simulink library "lib_transmission2"  (Simulink 10.1)
settings: Solver=VariableStepAuto  StartTime=0.0  StopTime=10.0  RelTol=1e-3
undefined symbols (not defined in the file or in its folder): cyc_mph, fc_map_spd, fc_max_trq, fc_spd_scale, fc_trq_scale, fd_inertia, fd_loss, fd_ratio, gb_gear_number_lookup, gb_gears_num, gb_inertia, gb_loss_const, gb_loss_input_spd_coeff, gb_loss_input_trq_coeff, gb_loss_output_spd_coeff, gb_loss_output_trq_coeff, gb_num_init, gb_ratio, gb_shift_delay, gb_spd_scale, gb_trq_scale, htc_inertia, htc_k_adv, htc_k_adv_coast, htc_lockup, htc_lockup_load, htc_lockup_spd, htc_lu_gear_range, htc_max_coast_tr, htc_min_coast_tr, htc_pump_loss_spd, htc_pump_loss_trq_lockup, htc_pump_loss_trq_unlock, htc_sr, htc_sr_coast, htc_tr, htc_tr_coast, htc_unlock_spd, mc_map_spd, mc_max_trq, mc_overtrq_factor, mc_spd_scale, mc_trq_scale, tc_loss, tc_mc_to_fc_ratio, tx_eff_map, tx_map_spd, tx_map_trq, tx_pg_r, tx_pg_s, tx_speed_dep, vc_clutch_bool, vc_idle_spd, vc_launch_spd, wh_radius
undefined symbols (not defined in the file): gb_dnshift_load, gb_dnshift_spd, gb_map_spd_out, gb_map_trq_in, gb_map_trq_out, gb_upshift_load, gb_upshift_spd, logFlag
libraries: lib_controls x1, lib_etc x1, lib_controls2 x1, lib_transmission x1
(part 11 of 17)

== system lib_transmission2/torque coupler <tc>/tc model & interface/tc model ==
  "torque and speed req'd at output side of torque coupler (Nm), (rad/s)" : Inport
  "torque and speed avail. at main input (Nm), (rad/s)" : Inport  Port=2
  "torque and speed avail. at motor input to tc (Nm), (rad/s)" : Inport  Port=3
  Block NOTES : Subsystem
      mask Display: disp('Block\nNOTES')
  Demux : Demux  Outputs=2
  Demux1 : Demux  Outputs=2
  Demux2 : Demux  Outputs=2
  MinMax : MinMax  Inputs=2
  MinMax1 : MinMax  Inputs=2
  Mux : Mux  Inputs=2
  Mux1 : Mux  Inputs=2
  Mux2 : Mux  Inputs=2
  Product : Product  Inputs=1  SaturateOnIntegerOverflow=on
  Product1 : Product  Inputs=1  SaturateOnIntegerOverflow=on
  effect of motor torque at output of tc (Nm) : Gain  Gain=tc_mc_to_fc_ratio  SaturateOnIntegerOverflow=on
  enhancedToWorkspace : Subsystem  TreatAsAtomicUnit=on  mask(enhancedToWorkspace){generalName=generalName, specificName=spd_out_r, logFlag=logFlag}
      mask prompts: generalName "General Name [char-evaluated]"; specificName "Specific Name [char-literal]"; logFlag "Enable flag (1=on,0=off)"
      mask help: A wrapper for the Simulink "To Workspace" block that allows you to evaluate the name of the variable to log to workspace. This is useful to avoid the double logging errors that occur when you pull in two library models that attempt to log to the same variable.
      mask init:
      | enhancedToWsMaker
      settings: CopyFcn=breakLinkCopyFcn  ParentCloseFcn=breakLinkParCloseFcn
      mask Help:
      | <h2>Enhanced To Workspace Block</h2>
      | <h3>Parameters</h3>
      | <UL>
      | <li><b>General Name:</b> This is the more general name of the variable. Variables are saved to the workspace as <i>generalName_specificName</i>. Note that this is an evaluated variable. If you would like to type in the value directly, it must be surrounded with single quotes. Otherwise you can input the name of a variable containing a char string.</li>
      | <li><b>Specific Name:</b> This is the specific name of the variable. Note that this is input as a char literal (i.e., you don't need quotes).</li>
      | <li><b>Enable Flag:</b> This flag should have the value of 0 or 1. If 0, the variable will not be logged to the workspace. If 1, the variable will be logged. This is done so that variable logging can be turned off to improve speed.</li>
      | </ul>
      | <h3>Overview</h3>
      | <p>The enhanced to workspace block was put together to allow one to dynamically resolve variable names at run time in simulink. This is most powerful when used in conjunction with a masked subsystem to allow multiple instances of that masked subsytem to be used in the same model. The strategy is to set the generalName in the block mask which will allow the block to change the general name for all variable logging on the fly.
      | <h3>Helper Files</h3>
      | <p>Three m-files are required by the enhancedToWorkspace block. These files are located in the &lt; ADVISOR root &gt;/GUI directory :
      | <ul>
      | <li><i>enhancedToWsMaker.m</i> This file runs the mask initialization for the block</li>
      | <li><i>breakLinkCopyFcn.m</i> This file is used by the block callback when the simulink block is copied. It is necessary to break the link to the enhancedToWorkspace similar to the To Workspace block in order for it to be able to configure itself. (Try copying simulink's To Workspace block--it is impossible to make a link)</li>
      | <li><i>breakLinkParCloseFcn.m</i> This file is similar to the breakLinkCopyFcn and is used when a parent system is closed</li>
      | </ul>
      | <hr>
      | 
      | <p>Created 2003-Jan-21, Michael Patrick O'Keefe, NREL</p>
      | 
      | <!--
      | <VARDEF>
      | <H3>var_name</H3>
      | <UL>
      | <LI><B>data type</B> data type here</LI>
      | <LI><B>units</B> units here</LI>
      | <LI><B>vehicle type</B> vehicle type here</LI>
      | <LI><B>description</B> description here</LI>
      | </UL>
      | </VARDEF>
      | -->
      mask Display: disp([generalName,'_',specificName])
  enhancedToWorkspace1 : Subsystem  TreatAsAtomicUnit=on  mask(enhancedToWorkspace){generalName=generalName, specificName=trq_out_r, logFlag=logFlag}
      mask prompts: generalName "General Name [char-evaluated]"; specificName "Specific Name [char-literal]"; logFlag "Enable flag (1=on,0=off)"
      mask help: A wrapper for the Simulink "To Workspace" block that allows you to evaluate the name of the variable to log to workspace. This is useful to avoid the double logging errors that occur when you pull in two library models that attempt to log to the same variable.
      mask init:
      | enhancedToWsMaker
      settings: CopyFcn=breakLinkCopyFcn  ParentCloseFcn=breakLinkParCloseFcn
      mask Help:
      | <h2>Enhanced To Workspace Block</h2>
      | <h3>Parameters</h3>
      | <UL>
      | <li><b>General Name:</b> This is the more general name of the variable. Variables are saved to the workspace as <i>generalName_specificName</i>. Note that this is an evaluated variable. If you would like to type in the value directly, it must be surrounded with single quotes. Otherwise you can input the name of a variable containing a char string.</li>
      | <li><b>Specific Name:</b> This is the specific name of the variable. Note that this is input as a char literal (i.e., you don't need quotes).</li>
      | <li><b>Enable Flag:</b> This flag should have the value of 0 or 1. If 0, the variable will not be logged to the workspace. If 1, the variable will be logged. This is done so that variable logging can be turned off to improve speed.</li>
      | </ul>
      | <h3>Overview</h3>
      | <p>The enhanced to workspace block was put together to allow one to dynamically resolve variable names at run time in simulink. This is most powerful when used in conjunction with a masked subsystem to allow multiple instances of that masked subsytem to be used in the same model. The strategy is to set the generalName in the block mask which will allow the block to change the general name for all variable logging on the fly.
      | <h3>Helper Files</h3>
      | <p>Three m-files are required by the enhancedToWorkspace block. These files are located in the &lt; ADVISOR root &gt;/GUI directory :
      | <ul>
      | <li><i>enhancedToWsMaker.m</i> This file runs the mask initialization for the block</li>
      | <li><i>breakLinkCopyFcn.m</i> This file is used by the block callback when the simulink block is copied. It is necessary to break the link to the enhancedToWorkspace similar to the To Workspace block in order for it to be able to configure itself. (Try copying simulink's To Workspace block--it is impossible to make a link)</li>
      | <li><i>breakLinkParCloseFcn.m</i> This file is similar to the breakLinkCopyFcn and is used when a parent system is closed</li>
      | </ul>
      | <hr>
      | 
      | <p>Created 2003-Jan-21, Michael Patrick O'Keefe, NREL</p>
      | 
      | <!--
      | <VARDEF>
      | <H3>var_name</H3>
      | <UL>
      | <LI><B>data type</B> data type here</LI>
      | <LI><B>units</B> units here</LI>
      | <LI><B>vehicle type</B> vehicle type here</LI>
      | <LI><B>description</B> description here</LI>
      | </UL>
      | </VARDEF>
      | -->
      mask Display: disp([generalName,'_',specificName])
  enhancedToWorkspace2 : Subsystem  TreatAsAtomicUnit=on  mask(enhancedToWorkspace){generalName=generalName, specificName=pwr_in_a, logFlag=logFlag}
      mask prompts: generalName "General Name [char-evaluated]"; specificName "Specific Name [char-literal]"; logFlag "Enable flag (1=on,0=off)"
      mask help: A wrapper for the Simulink "To Workspace" block that allows you to evaluate the name of the variable to log to workspace. This is useful to avoid the double logging errors that occur when you pull in two library models that attempt to log to the same variable.
      mask init:
      | enhancedToWsMaker
      settings: CopyFcn=breakLinkCopyFcn  ParentCloseFcn=breakLinkParCloseFcn
      mask Help:
      | <h2>Enhanced To Workspace Block</h2>
      | <h3>Parameters</h3>
      | <UL>
      | <li><b>General Name:</b> This is the more general name of the variable. Variables are saved to the workspace as <i>generalName_specificName</i>. Note that this is an evaluated variable. If you would like to type in the value directly, it must be surrounded with single quotes. Otherwise you can input the name of a variable containing a char string.</li>
      | <li><b>Specific Name:</b> This is the specific name of the variable. Note that this is input as a char literal (i.e., you don't need quotes).</li>
      | <li><b>Enable Flag:</b> This flag should have the value of 0 or 1. If 0, the variable will not be logged to the workspace. If 1, the variable will be logged. This is done so that variable logging can be turned off to improve speed.</li>
      | </ul>
      | <h3>Overview</h3>
      | <p>The enhanced to workspace block was put together to allow one to dynamically resolve variable names at run time in simulink. This is most powerful when used in conjunction with a masked subsystem to allow multiple instances of that masked subsytem to be used in the same model. The strategy is to set the generalName in the block mask which will allow the block to change the general name for all variable logging on the fly.
      | <h3>Helper Files</h3>
      | <p>Three m-files are required by the enhancedToWorkspace block. These files are located in the &lt; ADVISOR root &gt;/GUI directory :
      | <ul>
      | <li><i>enhancedToWsMaker.m</i> This file runs the mask initialization for the block</li>
      | <li><i>breakLinkCopyFcn.m</i> This file is used by the block callback when the simulink block is copied. It is necessary to break the link to the enhancedToWorkspace similar to the To Workspace block in order for it to be able to configure itself. (Try copying simulink's To Workspace block--it is impossible to make a link)</li>
      | <li><i>breakLinkParCloseFcn.m</i> This file is similar to the breakLinkCopyFcn and is used when a parent system is closed</li>
      | </ul>
      | <hr>
      | 
      | <p>Created 2003-Jan-21, Michael Patrick O'Keefe, NREL</p>
      | 
      | <!--
      | <VARDEF>
      | <H3>var_name</H3>
      | <UL>
      | <LI><B>data type</B> data type here</LI>
      | <LI><B>units</B> units here</LI>
      | <LI><B>vehicle type</B> vehicle type here</LI>
      | <LI><B>description</B> description here</LI>
      | </UL>
      | </VARDEF>
      | -->
      mask Display: disp([generalName,'_',specificName])
  enhancedToWorkspace3 : Subsystem  TreatAsAtomicUnit=on  mask(enhancedToWorkspace){generalName=generalName, specificName=trq_out_a, logFlag=logFlag}
      mask prompts: generalName "General Name [char-evaluated]"; specificName "Specific Name [char-literal]"; logFlag "Enable flag (1=on,0=off)"
      mask help: A wrapper for the Simulink "To Workspace" block that allows you to evaluate the name of the variable to log to workspace. This is useful to avoid the double logging errors that occur when you pull in two library models that attempt to log to the same variable.
      mask init:
      | enhancedToWsMaker
      settings: CopyFcn=breakLinkCopyFcn  ParentCloseFcn=breakLinkParCloseFcn
      mask Help:
      | <h2>Enhanced To Workspace Block</h2>
      | <h3>Parameters</h3>
      | <UL>
      | <li><b>General Name:</b> This is the more general name of the variable. Variables are saved to the workspace as <i>generalName_specificName</i>. Note that this is an evaluated variable. If you would like to type in the value directly, it must be surrounded with single quotes. Otherwise you can input the name of a variable containing a char string.</li>
      | <li><b>Specific Name:</b> This is the specific name of the variable. Note that this is input as a char literal (i.e., you don't need quotes).</li>
      | <li><b>Enable Flag:</b> This flag should have the value of 0 or 1. If 0, the variable will not be logged to the workspace. If 1, the variable will be logged. This is done so that variable logging can be turned off to improve speed.</li>
      | </ul>
      | <h3>Overview</h3>
      | <p>The enhanced to workspace block was put together to allow one to dynamically resolve variable names at run time in simulink. This is most powerful when used in conjunction with a masked subsystem to allow multiple instances of that masked subsytem to be used in the same model. The strategy is to set the generalName in the block mask which will allow the block to change the general name for all variable logging on the fly.
      | <h3>Helper Files</h3>
      | <p>Three m-files are required by the enhancedToWorkspace block. These files are located in the &lt; ADVISOR root &gt;/GUI directory :
      | <ul>
      | <li><i>enhancedToWsMaker.m</i> This file runs the mask initialization for the block</li>
      | <li><i>breakLinkCopyFcn.m</i> This file is used by the block callback when the simulink block is copied. It is necessary to break the link to the enhancedToWorkspace similar to the To Workspace block in order for it to be able to configure itself. (Try copying simulink's To Workspace block--it is impossible to make a link)</li>
      | <li><i>breakLinkParCloseFcn.m</i> This file is similar to the breakLinkCopyFcn and is used when a parent system is closed</li>
      | </ul>
      | <hr>
      | 
      | <p>Created 2003-Jan-21, Michael Patrick O'Keefe, NREL</p>
      | 
      | <!--
      | <VARDEF>
      | <H3>var_name</H3>
      | <UL>
      | <LI><B>data type</B> data type here</LI>
      | <LI><B>units</B> units here</LI>
      | <LI><B>vehicle type</B> vehicle type here</LI>
      | <LI><B>description</B> description here</LI>
      | </UL>
      | </VARDEF>
      | -->
      mask Display: disp([generalName,'_',specificName])
  enhancedToWorkspace4 : Subsystem  TreatAsAtomicUnit=on  mask(enhancedToWorkspace){generalName=generalName, specificName=spd_out_a, logFlag=logFlag}
      mask prompts: generalName "General Name [char-evaluated]"; specificName "Specific Name [char-literal]"; logFlag "Enable flag (1=on,0=off)"
      mask help: A wrapper for the Simulink "To Workspace" block that allows you to evaluate the name of the variable to log to workspace. This is useful to avoid the double logging errors that occur when you pull in two library models that attempt to log to the same variable.
      mask init:
      | enhancedToWsMaker
      settings: CopyFcn=breakLinkCopyFcn  ParentCloseFcn=breakLinkParCloseFcn
      mask Help:
      | <h2>Enhanced To Workspace Block</h2>
      | <h3>Parameters</h3>
      | <UL>
      | <li><b>General Name:</b> This is the more general name of the variable. Variables are saved to the workspace as <i>generalName_specificName</i>. Note that this is an evaluated variable. If you would like to type in the value directly, it must be surrounded with single quotes. Otherwise you can input the name of a variable containing a char string.</li>
      | <li><b>Specific Name:</b> This is the specific name of the variable. Note that this is input as a char literal (i.e., you don't need quotes).</li>
      | <li><b>Enable Flag:</b> This flag should have the value of 0 or 1. If 0, the variable will not be logged to the workspace. If 1, the variable will be logged. This is done so that variable logging can be turned off to improve speed.</li>
      | </ul>
      | <h3>Overview</h3>
      | <p>The enhanced to workspace block was put together to allow one to dynamically resolve variable names at run time in simulink. This is most powerful when used in conjunction with a masked subsystem to allow multiple instances of that masked subsytem to be used in the same model. The strategy is to set the generalName in the block mask which will allow the block to change the general name for all variable logging on the fly.
      | <h3>Helper Files</h3>
      | <p>Three m-files are required by the enhancedToWorkspace block. These files are located in the &lt; ADVISOR root &gt;/GUI directory :
      | <ul>
      | <li><i>enhancedToWsMaker.m</i> This file runs the mask initialization for the block</li>
      | <li><i>breakLinkCopyFcn.m</i> This file is used by the block callback when the simulink block is copied. It is necessary to break the link to the enhancedToWorkspace similar to the To Workspace block in order for it to be able to configure itself. (Try copying simulink's To Workspace block--it is impossible to make a link)</li>
      | <li><i>breakLinkParCloseFcn.m</i> This file is similar to the breakLinkCopyFcn and is used when a parent system is closed</li>
      | </ul>
      | <hr>
      | 
      | <p>Created 2003-Jan-21, Michael Patrick O'Keefe, NREL</p>
      | 
      | <!--
      | <VARDEF>
      | <H3>var_name</H3>
      | <UL>
      | <LI><B>data type</B> data type here</LI>
      | <LI><B>units</B> units here</LI>
      | <LI><B>vehicle type</B> vehicle type here</LI>
      | <LI><B>description</B> description here</LI>
      | </UL>
      | </VARDEF>
      | -->
      mask Display: disp([generalName,'_',specificName])
  help : Subsystem
      settings: OpenFcn=web(['file:\\\' which('torque_coupler.htm')]);
      mask Display: image(imread('doc_man.jpg'))
  loss (Nm) : Subsystem
  speed of output gear corresponding to motor spd (rad/s) : Gain  Gain=1/tc_mc_to_fc_ratio  SaturateOnIntegerOverflow=on
  speed req'd of motor (rad/s) : Gain  Gain=tc_mc_to_fc_ratio  SaturateOnIntegerOverflow=on
  "sum " : Sum  SaturateOnIntegerOverflow=on
  torque avail. at output side of tc (Nm) : Sum  Inputs=-++  SaturateOnIntegerOverflow=on
  total torque req'd at output gear (Nm) : Sum  SaturateOnIntegerOverflow=on
  total torque req'd of motor (Nm) : Gain  Gain=1/tc_mc_to_fc_ratio  SaturateOnIntegerOverflow=on
  unmet torque request (Nm) : Sum  Inputs=+-  SaturateOnIntegerOverflow=on
  "torque and speed req'd at main input to torque coupler (Nm), (rad/s)" : Outport  InitialOutput=0
  "torque and speed req'd at motor input to torque coupler (Nm), (rad/s)" : Outport  Port=2  InitialOutput=0
  "torque and speed avail. at output side of torque coupler (Nm), (rad/s)" : Outport  Port=3  InitialOutput=0
  wires:
  MinMax1/1 -> Mux2/2, enhancedToWorkspace4/1(In1)
  torque avail. at output side of tc (Nm)/1 -> Mux2/1, enhancedToWorkspace3/1(In1)
  Demux/1 -> total torque req'd at output gear (Nm)/1, enhancedToWorkspace1/1(In1)
  MinMax/1 -> MinMax1/1, speed req'd of motor (rad/s)/1
  speed of output gear corresponding to motor spd (rad/s)/1 -> MinMax1/2
  Demux2/2 -> speed of output gear corresponding to motor spd (rad/s)/1
  Mux2/1 -> "torque and speed avail. at output side of torque coupler (Nm), (rad/s)"/1
  effect of motor torque at output of tc (Nm)/1 -> torque avail. at output side of tc (Nm)/3
  Demux2/1 -> effect of motor torque at output of tc (Nm)/1
  Demux1/1 -> torque avail. at output side of tc (Nm)/2, unmet torque request (Nm)/2
  loss (Nm)/1(drag torque (Nm)) -> torque avail. at output side of tc (Nm)/1, total torque req'd at output gear (Nm)/2
  speed req'd of motor (rad/s)/1 -> Mux1/2
  total torque req'd of motor (Nm)/1 -> Mux1/1
  Mux1/1 -> "torque and speed req'd at motor input to torque coupler (Nm), (rad/s)"/1
  Demux1/2 -> MinMax/2
  unmet torque request (Nm)/1 -> total torque req'd of motor (Nm)/1
  total torque req'd at output gear (Nm)/1 -> unmet torque request (Nm)/1, Mux/1
  Demux/2 -> MinMax/1, enhancedToWorkspace/1(In1), Mux/2, loss (Nm)/1(tc output speed (rad/s))
  "torque and speed req'd at output side of torque coupler (Nm), (rad/s)"/1 -> Demux/1
  Mux/1 -> "torque and speed req'd at main input to torque coupler (Nm), (rad/s)"/1
  "sum "/1 -> enhancedToWorkspace2/1(In1)
  Product/1 -> "sum "/1
  "torque and speed avail. at main input (Nm), (rad/s)"/1 -> Demux1/1, Product/1
  "torque and speed avail. at motor input to tc (Nm), (rad/s)"/1 -> Demux2/1, Product1/1
  Product1/1 -> "sum "/2

== system lib_transmission2/torque coupler <tc> DIRECT SPLIT/tc direct split model & interface/signal annotator ==
  In1 : Inport
  Demux : Demux  Outputs=2
  Mux : Mux  Inputs=2
  Out1 : Outport
  wires:
  In1/1 -> Demux/1
  Demux/1 -> Mux/1  "tc_trq_out_r"
  Demux/2 -> Mux/2  "tc_spd_out_r"
  Mux/1 -> Out1/1

== system lib_transmission2/torque coupler <tc> DIRECT SPLIT/tc direct split model & interface/tc direct split model ==
  note: FOR THE HONDA INSIGHT
      | Since both the Electric Motor and the IC Engine are on the same shaft,
      | there is no actual torque coupler. Thus, this is a hypothetical torque coupler used for
      | generality, with a transmission ratio of 1 (The variable is tc_mc_to_fc_ratio),
      | with zero losses. In case this model is used for any other configuration, losses
      | and a ratio may be added.
  note: Ratio = 1 for the HONDA INSIGHT
  note: Torque
  note: Speed
  "torque and speed req'd at output side of torque coupler (Nm), (rad/s)" : Inport
  "torque and speed avail. at main input (Nm), (rad/s)" : Inport  Port=2
  "torque and speed avail. at motor input to tc (Nm), (rad/s)" : Inport  Port=3
  Block NOTES : Subsystem
      mask Display: disp('Block\nNOTES')
  Demux : Demux  Outputs=2
  Demux1 : Demux  Outputs=2
  Demux2 : Demux  Outputs=2
  MinMax : MinMax  Inputs=2
  MinMax1 : MinMax  Inputs=2
  Mux : Mux  Inputs=2
  Mux2 : Mux  Inputs=2
  Product : Product  Inputs=1  SaturateOnIntegerOverflow=on
  Product1 : Product  Inputs=1  SaturateOnIntegerOverflow=on
  effect of motor torque at output of tc (Nm) : Gain  Gain=tc_mc_to_fc_ratio  SaturateOnIntegerOverflow=on
  enhancedToWorkspace : Subsystem  TreatAsAtomicUnit=on  mask(enhancedToWorkspace){generalName=generalName, specificName=trq_out_r, logFlag=logFlag}
      mask prompts: generalName "General Name [char-evaluated]"; specificName "Specific Name [char-literal]"; logFlag "Enable flag (1=on,0=off)"
      mask help: A wrapper for the Simulink "To Workspace" block that allows you to evaluate the name of the variable to log to workspace. This is useful to avoid the double logging errors that occur when you pull in two library models that attempt to log to the same variable.
      mask init:
      | enhancedToWsMaker
      settings: CopyFcn=breakLinkCopyFcn  ParentCloseFcn=breakLinkParCloseFcn
      mask Help:
      | <h2>Enhanced To Workspace Block</h2>
      | <h3>Parameters</h3>
      | <UL>
      | <li><b>General Name:</b> This is the more general name of the variable. Variables are saved to the workspace as <i>generalName_specificName</i>. Note that this is an evaluated variable. If you would like to type in the value directly, it must be surrounded with single quotes. Otherwise you can input the name of a variable containing a char string.</li>
      | <li><b>Specific Name:</b> This is the specific name of the variable. Note that this is input as a char literal (i.e., you don't need quotes).</li>
      | <li><b>Enable Flag:</b> This flag should have the value of 0 or 1. If 0, the variable will not be logged to the workspace. If 1, the variable will be logged. This is done so that variable logging can be turned off to improve speed.</li>
      | </ul>
      | <h3>Overview</h3>
      | <p>The enhanced to workspace block was put together to allow one to dynamically resolve variable names at run time in simulink. This is most powerful when used in conjunction with a masked subsystem to allow multiple instances of that masked subsytem to be used in the same model. The strategy is to set the generalName in the block mask which will allow the block to change the general name for all variable logging on the fly.
      | <h3>Helper Files</h3>
      | <p>Three m-files are required by the enhancedToWorkspace block. These files are located in the &lt; ADVISOR root &gt;/GUI directory :
      | <ul>
      | <li><i>enhancedToWsMaker.m</i> This file runs the mask initialization for the block</li>
      | <li><i>breakLinkCopyFcn.m</i> This file is used by the block callback when the simulink block is copied. It is necessary to break the link to the enhancedToWorkspace similar to the To Workspace block in order for it to be able to configure itself. (Try copying simulink's To Workspace block--it is impossible to make a link)</li>
      | <li><i>breakLinkParCloseFcn.m</i> This file is similar to the breakLinkCopyFcn and is used when a parent system is closed</li>
      | </ul>
      | <hr>
      | 
      | <p>Created 2003-Jan-21, Michael Patrick O'Keefe, NREL</p>
      | 
      | <!--
      | <VARDEF>
      | <H3>var_name</H3>
      | <UL>
      | <LI><B>data type</B> data type here</LI>
      | <LI><B>units</B> units here</LI>
      | <LI><B>vehicle type</B> vehicle type here</LI>
      | <LI><B>description</B> description here</LI>
      | </UL>
      | </VARDEF>
      | -->
      mask Display: disp([generalName,'_',specificName])
  enhancedToWorkspace1 : Subsystem  TreatAsAtomicUnit=on  mask(enhancedToWorkspace){generalName=generalName, specificName=spd_out_r, logFlag=logFlag}
      mask prompts: generalName "General Name [char-evaluated]"; specificName "Specific Name [char-literal]"; logFlag "Enable flag (1=on,0=off)"
      mask help: A wrapper for the Simulink "To Workspace" block that allows you to evaluate the name of the variable to log to workspace. This is useful to avoid the double logging errors that occur when you pull in two library models that attempt to log to the same variable.
      mask init:
      | enhancedToWsMaker
      settings: CopyFcn=breakLinkCopyFcn  ParentCloseFcn=breakLinkParCloseFcn
      mask Help:
      | <h2>Enhanced To Workspace Block</h2>
      | <h3>Parameters</h3>
      | <UL>
      | <li><b>General Name:</b> This is the more general name of the variable. Variables are saved to the workspace as <i>generalName_specificName</i>. Note that this is an evaluated variable. If you would like to type in the value directly, it must be surrounded with single quotes. Otherwise you can input the name of a variable containing a char string.</li>
      | <li><b>Specific Name:</b> This is the specific name of the variable. Note that this is input as a char literal (i.e., you don't need quotes).</li>
      | <li><b>Enable Flag:</b> This flag should have the value of 0 or 1. If 0, the variable will not be logged to the workspace. If 1, the variable will be logged. This is done so that variable logging can be turned off to improve speed.</li>
      | </ul>
      | <h3>Overview</h3>
      | <p>The enhanced to workspace block was put together to allow one to dynamically resolve variable names at run time in simulink. This is most powerful when used in conjunction with a masked subsystem to allow multiple instances of that masked subsytem to be used in the same model. The strategy is to set the generalName in the block mask which will allow the block to change the general name for all variable logging on the fly.
      | <h3>Helper Files</h3>
      | <p>Three m-files are required by the enhancedToWorkspace block. These files are located in the &lt; ADVISOR root &gt;/GUI directory :
      | <ul>
      | <li><i>enhancedToWsMaker.m</i> This file runs the mask initialization for the block</li>
      | <li><i>breakLinkCopyFcn.m</i> This file is used by the block callback when the simulink block is copied. It is necessary to break the link to the enhancedToWorkspace similar to the To Workspace block in order for it to be able to configure itself. (Try copying simulink's To Workspace block--it is impossible to make a link)</li>
      | <li><i>breakLinkParCloseFcn.m</i> This file is similar to the breakLinkCopyFcn and is used when a parent system is closed</li>
      | </ul>
      | <hr>
      | 
      | <p>Created 2003-Jan-21, Michael Patrick O'Keefe, NREL</p>
      | 
      | <!--
      | <VARDEF>
      | <H3>var_name</H3>
      | <UL>
      | <LI><B>data type</B> data type here</LI>
      | <LI><B>units</B> units here</LI>
      | <LI><B>vehicle type</B> vehicle type here</LI>
      | <LI><B>description</B> description here</LI>
      | </UL>
      | </VARDEF>
      | -->
      mask Display: disp([generalName,'_',specificName])
  enhancedToWorkspace2 : Subsystem  TreatAsAtomicUnit=on  mask(enhancedToWorkspace){generalName=generalName, specificName=pwr_in_a, logFlag=logFlag}
      mask prompts: generalName "General Name [char-evaluated]"; specificName "Specific Name [char-literal]"; logFlag "Enable flag (1=on,0=off)"
      mask help: A wrapper for the Simulink "To Workspace" block that allows you to evaluate the name of the variable to log to workspace. This is useful to avoid the double logging errors that occur when you pull in two library models that attempt to log to the same variable.
      mask init:
      | enhancedToWsMaker
      settings: CopyFcn=breakLinkCopyFcn  ParentCloseFcn=breakLinkParCloseFcn
      mask Help:
      | <h2>Enhanced To Workspace Block</h2>
      | <h3>Parameters</h3>
      | <UL>
      | <li><b>General Name:</b> This is the more general name of the variable. Variables are saved to the workspace as <i>generalName_specificName</i>. Note that this is an evaluated variable. If you would like to type in the value directly, it must be surrounded with single quotes. Otherwise you can input the name of a variable containing a char string.</li>
      | <li><b>Specific Name:</b> This is the specific name of the variable. Note that this is input as a char literal (i.e., you don't need quotes).</li>
      | <li><b>Enable Flag:</b> This flag should have the value of 0 or 1. If 0, the variable will not be logged to the workspace. If 1, the variable will be logged. This is done so that variable logging can be turned off to improve speed.</li>
      | </ul>
      | <h3>Overview</h3>
      | <p>The enhanced to workspace block was put together to allow one to dynamically resolve variable names at run time in simulink. This is most powerful when used in conjunction with a masked subsystem to allow multiple instances of that masked subsytem to be used in the same model. The strategy is to set the generalName in the block mask which will allow the block to change the general name for all variable logging on the fly.
      | <h3>Helper Files</h3>
      | <p>Three m-files are required by the enhancedToWorkspace block. These files are located in the &lt; ADVISOR root &gt;/GUI directory :
      | <ul>
      | <li><i>enhancedToWsMaker.m</i> This file runs the mask initialization for the block</li>
      | <li><i>breakLinkCopyFcn.m</i> This file is used by the block callback when the simulink block is copied. It is necessary to break the link to the enhancedToWorkspace similar to the To Workspace block in order for it to be able to configure itself. (Try copying simulink's To Workspace block--it is impossible to make a link)</li>
      | <li><i>breakLinkParCloseFcn.m</i> This file is similar to the breakLinkCopyFcn and is used when a parent system is closed</li>
      | </ul>
      | <hr>
      | 
      | <p>Created 2003-Jan-21, Michael Patrick O'Keefe, NREL</p>
      | 
      | <!--
      | <VARDEF>
      | <H3>var_name</H3>
      | <UL>
      | <LI><B>data type</B> data type here</LI>
      | <LI><B>units</B> units here</LI>
      | <LI><B>vehicle type</B> vehicle type here</LI>
      | <LI><B>description</B> description here</LI>
      | </UL>
      | </VARDEF>
      | -->
      mask Display: disp([generalName,'_',specificName])
  enhancedToWorkspace3 : Subsystem  TreatAsAtomicUnit=on  mask(enhancedToWorkspace){generalName=generalName, specificName=spd_out_a, logFlag=logFlag}
      mask prompts: generalName "General Name [char-evaluated]"; specificName "Specific Name [char-literal]"; logFlag "Enable flag (1=on,0=off)"
      mask help: A wrapper for the Simulink "To Workspace" block that allows you to evaluate the name of the variable to log to workspace. This is useful to avoid the double logging errors that occur when you pull in two library models that attempt to log to the same variable.
      mask init:
      | enhancedToWsMaker
      settings: CopyFcn=breakLinkCopyFcn  ParentCloseFcn=breakLinkParCloseFcn
      mask Help:
      | <h2>Enhanced To Workspace Block</h2>
      | <h3>Parameters</h3>
      | <UL>
      | <li><b>General Name:</b> This is the more general name of the variable. Variables are saved to the workspace as <i>generalName_specificName</i>. Note that this is an evaluated variable. If you would like to type in the value directly, it must be surrounded with single quotes. Otherwise you can input the name of a variable containing a char string.</li>
      | <li><b>Specific Name:</b> This is the specific name of the variable. Note that this is input as a char literal (i.e., you don't need quotes).</li>
      | <li><b>Enable Flag:</b> This flag should have the value of 0 or 1. If 0, the variable will not be logged to the workspace. If 1, the variable will be logged. This is done so that variable logging can be turned off to improve speed.</li>
      | </ul>
      | <h3>Overview</h3>
      | <p>The enhanced to workspace block was put together to allow one to dynamically resolve variable names at run time in simulink. This is most powerful when used in conjunction with a masked subsystem to allow multiple instances of that masked subsytem to be used in the same model. The strategy is to set the generalName in the block mask which will allow the block to change the general name for all variable logging on the fly.
      | <h3>Helper Files</h3>
      | <p>Three m-files are required by the enhancedToWorkspace block. These files are located in the &lt; ADVISOR root &gt;/GUI directory :
      | <ul>
      | <li><i>enhancedToWsMaker.m</i> This file runs the mask initialization for the block</li>
      | <li><i>breakLinkCopyFcn.m</i> This file is used by the block callback when the simulink block is copied. It is necessary to break the link to the enhancedToWorkspace similar to the To Workspace block in order for it to be able to configure itself. (Try copying simulink's To Workspace block--it is impossible to make a link)</li>
      | <li><i>breakLinkParCloseFcn.m</i> This file is similar to the breakLinkCopyFcn and is used when a parent system is closed</li>
      | </ul>
      | <hr>
      | 
      | <p>Created 2003-Jan-21, Michael Patrick O'Keefe, NREL</p>
      | 
      | <!--
      | <VARDEF>
      | <H3>var_name</H3>
      | <UL>
      | <LI><B>data type</B> data type here</LI>
      | <LI><B>units</B> units here</LI>
      | <LI><B>vehicle type</B> vehicle type here</LI>
      | <LI><B>description</B> description here</LI>
      | </UL>
      | </VARDEF>
      | -->
      mask Display: disp([generalName,'_',specificName])
  enhancedToWorkspace4 : Subsystem  TreatAsAtomicUnit=on  mask(enhancedToWorkspace){generalName=generalName, specificName=trq_out_a, logFlag=logFlag}
      mask prompts: generalName "General Name [char-evaluated]"; specificName "Specific Name [char-literal]"; logFlag "Enable flag (1=on,0=off)"
      mask help: A wrapper for the Simulink "To Workspace" block that allows you to evaluate the name of the variable to log to workspace. This is useful to avoid the double logging errors that occur when you pull in two library models that attempt to log to the same variable.
      mask init:
      | enhancedToWsMaker
      settings: CopyFcn=breakLinkCopyFcn  ParentCloseFcn=breakLinkParCloseFcn
      mask Help:
      | <h2>Enhanced To Workspace Block</h2>
      | <h3>Parameters</h3>
      | <UL>
      | <li><b>General Name:</b> This is the more general name of the variable. Variables are saved to the workspace as <i>generalName_specificName</i>. Note that this is an evaluated variable. If you would like to type in the value directly, it must be surrounded with single quotes. Otherwise you can input the name of a variable containing a char string.</li>
      | <li><b>Specific Name:</b> This is the specific name of the variable. Note that this is input as a char literal (i.e., you don't need quotes).</li>
      | <li><b>Enable Flag:</b> This flag should have the value of 0 or 1. If 0, the variable will not be logged to the workspace. If 1, the variable will be logged. This is done so that variable logging can be turned off to improve speed.</li>
      | </ul>
      | <h3>Overview</h3>
      | <p>The enhanced to workspace block was put together to allow one to dynamically resolve variable names at run time in simulink. This is most powerful when used in conjunction with a masked subsystem to allow multiple instances of that masked subsytem to be used in the same model. The strategy is to set the generalName in the block mask which will allow the block to change the general name for all variable logging on the fly.
      | <h3>Helper Files</h3>
      | <p>Three m-files are required by the enhancedToWorkspace block. These files are located in the &lt; ADVISOR root &gt;/GUI directory :
      | <ul>
      | <li><i>enhancedToWsMaker.m</i> This file runs the mask initialization for the block</li>
      | <li><i>breakLinkCopyFcn.m</i> This file is used by the block callback when the simulink block is copied. It is necessary to break the link to the enhancedToWorkspace similar to the To Workspace block in order for it to be able to configure itself. (Try copying simulink's To Workspace block--it is impossible to make a link)</li>
      | <li><i>breakLinkParCloseFcn.m</i> This file is similar to the breakLinkCopyFcn and is used when a parent system is closed</li>
      | </ul>
      | <hr>
      | 
      | <p>Created 2003-Jan-21, Michael Patrick O'Keefe, NREL</p>
      | 
      | <!--
      | <VARDEF>
      | <H3>var_name</H3>
      | <UL>
      | <LI><B>data type</B> data type here</LI>
      | <LI><B>units</B> units here</LI>
      | <LI><B>vehicle type</B> vehicle type here</LI>
      | <LI><B>description</B> description here</LI>
      | </UL>
      | </VARDEF>
      | -->
      mask Display: disp([generalName,'_',specificName])
  help : Subsystem
      settings: OpenFcn=web(['file:\\\' which('torque_coupler.htm')]);
      mask Display: image(imread('doc_man.jpg'))
  loss (Nm) : Subsystem
  speed of output gear corresponding to motor spd (rad/s) : Gain  Gain=1/tc_mc_to_fc_ratio  SaturateOnIntegerOverflow=on
  "sum " : Sum  SaturateOnIntegerOverflow=on
  torque avail. at output side of tc (Nm) : Sum  SaturateOnIntegerOverflow=on
  total torque req'd at output gear (Nm) Loss==0 for the INSIGHT : Sum  SaturateOnIntegerOverflow=on
  "torque and speed req'd at main input to torque coupler (Nm), (rad/s)" : Outport  InitialOutput=0
  "torque and speed avail. at output side of torque coupler (Nm), (rad/s)" : Outport  Port=2  InitialOutput=0
  wires:
  MinMax1/1 -> Mux2/2, enhancedToWorkspace3/1(In1)
  speed of output gear corresponding to motor spd (rad/s)/1 -> MinMax1/2
  Demux2/2 -> speed of output gear corresponding to motor spd (rad/s)/1
  effect of motor torque at output of tc (Nm)/1 -> torque avail. at output side of tc (Nm)/2
  Demux2/1 -> effect of motor torque at output of tc (Nm)/1
  Demux1/2 -> MinMax/2
  "torque and speed req'd at output side of torque coupler (Nm), (rad/s)"/1 -> Demux/1
  Mux/1 -> "torque and speed req'd at main input to torque coupler (Nm), (rad/s)"/1
  "sum "/1 -> enhancedToWorkspace2/1(In1)
  Product/1 -> "sum "/1
  "torque and speed avail. at main input (Nm), (rad/s)"/1 -> Demux1/1, Product/1
  "torque and speed avail. at motor input to tc (Nm), (rad/s)"/1 -> Demux2/1, Product1/1
  Product1/1 -> "sum "/2
  Demux1/1 -> torque avail. at output side of tc (Nm)/1
  MinMax/1 -> MinMax1/1
  Mux2/1 -> "torque and speed avail. at output side of torque coupler (Nm), (rad/s)"/1
  torque avail. at output side of tc (Nm)/1 -> Mux2/1, enhancedToWorkspace4/1(In1)
  Demux/2 -> MinMax/1, enhancedToWorkspace1/1(In1), loss (Nm)/1(tc output speed (rad/s)), Mux/2
  Demux/1 -> total torque req'd at output gear (Nm) Loss==0 for the INSIGHT/1, enhancedToWorkspace/1(In1)
  loss (Nm)/1(drag torque (Nm)) -> total torque req'd at output gear (Nm) Loss==0 for the INSIGHT/2
  total torque req'd at output gear (Nm) Loss==0 for the INSIGHT/1 -> Mux/1

== system lib_transmission2/Clutch Control/Clutch Control/Clutch Control/clutch control ==
  shifting : Inport
  gb_trq_in_r : Inport  Port=2
  gb_spd_in_r : Inport  Port=3
  Block NOTES : Subsystem
      mask Display: disp('Block\nNOTES')
  Constant : Constant  Value=1e-3
  Constant1 : Constant  Value=vc_clutch_bool
  Constant2 : Constant  Value=vc_idle_spd
  Constant3 : Constant  Value=1e-3
  Constant4 : Constant  Value=vc_launch_spd
  Constant5 : Constant  Value=2.5
  Fcn: 1 if clutch disengaged 2 if clutch slipping 3 if clutch engaged : Fcn  Expr=u[1]+2*u[2]*(1-u[1])*(1-u[3])+3*u[3]*(1-u[1])
  Logical Operator : Logic
  Logical Operator1 : Logic  Operator=OR
  Memory : Memory  InitialCondition=1+(2*(cyc_mph(1,2)>0))
  Mux : Mux  Inputs=3
  Relational Operator : RelationalOperator  Operator=<=  RndMeth=Nearest  InputSameDT=on
  Relational Operator1 : RelationalOperator  Operator=<  RndMeth=Nearest  InputSameDT=on
  Relational Operator2 : RelationalOperator  Operator=>  RndMeth=Nearest  InputSameDT=on
  Relational Operator3 : RelationalOperator  Operator=<  RndMeth=Nearest  InputSameDT=on
  clutch disengaged : Logic  Operator=OR
  clutch engaged : Logic  Operator=NOR
  clutch slipping : Logic  Inputs=3
  clutch was NOT fully engaged during last time step : RelationalOperator  Operator=<  RndMeth=Nearest  InputSameDT=on
  gearbox speed estimator : Subsystem
  clutch state : Outport
  wires:
  gearbox speed estimator/1(Out1) -> Relational Operator3/1, Relational Operator1/1
  gb_spd_in_r/1 -> gearbox speed estimator/1(gb_spd_in_r if no gear change)
  shifting/1 -> clutch disengaged/1
  Logical Operator/1 -> clutch disengaged/2
  gb_trq_in_r/1 -> Relational Operator2/1, Relational Operator/1
  Logical Operator1/1 -> Logical Operator/2
  Relational Operator/1 -> Logical Operator/1
  Constant/1 -> Relational Operator/2
  Constant1/1 -> Logical Operator1/1
  clutch was NOT fully engaged during last time step/1 -> clutch slipping/3
  Constant5/1 -> clutch was NOT fully engaged during last time step/2
  Memory/1 -> clutch was NOT fully engaged during last time step/1
  Relational Operator3/1 -> clutch slipping/2
  Constant4/1 -> Relational Operator3/2
  clutch slipping/1 -> Mux/2, clutch engaged/2
  Relational Operator2/1 -> clutch slipping/1
  Constant3/1 -> Relational Operator2/2
  Fcn: 1 if clutch disengaged 2 if clutch slipping 3 if clutch engaged/1 -> Memory/1, clutch state/1
  clutch disengaged/1 -> Mux/1, clutch engaged/1
  clutch engaged/1 -> Mux/3
  Mux/1 -> Fcn: 1 if clutch disengaged 2 if clutch slipping 3 if clutch engaged/1
  Constant2/1 -> Relational Operator1/2
  Relational Operator1/1 -> Logical Operator1/2

== system lib_transmission2/Clutch Control/Clutch Control/Clutch Control/repeated cycle:  speed required at end of NEXT step ==
  Clock : Clock
  Fcn1 : Fcn  Expr=rem(u[1],period)
  Look-Up Table : Lookup  InputValues=t  Table=y  SaturateOnIntegerOverflow=on
  Memory : Memory  InitialCondition=-0.1
  Sum : Sum  Inputs=+-  SaturateOnIntegerOverflow=on
  Sum1 : Sum  SaturateOnIntegerOverflow=on
  out_1 : Outport  InitialOutput=0
  wires:
  Clock/1 -> Sum/1, Memory/1, Fcn1/1
  Memory/1 -> Sum/2
  Sum/1 -> Sum1/2
  Fcn1/1 -> Sum1/1
  Look-Up Table/1 -> out_1/1
  Sum1/1 -> Look-Up Table/1

== system lib_transmission2/Gearbox Control/Gearbox Control manual shift logic/manual shift logic/gearbox  control ==
  note: local GOTO blocks:
  gb_trq_out_r : Inport
  gb_spd_out_r : Inport  Port=2
  prev. Pout/Pin : Inport  Port=3
  tires are at traction limit : Inport  Port=4
  Block NOTES : Subsystem
      mask Display: disp('Block\nNOTES')
  Constant : Constant
  Fcn : Fcn  Expr=1/u
  Fcn1 : Fcn  Expr=1/u
  Gain1 : Gain  Gain=-1  SaturateOnIntegerOverflow=on
  Product2 : Product  Inputs=*/  SaturateOnIntegerOverflow=on
  Product3 : Product  SaturateOnIntegerOverflow=on
  Rate Limiter : RateLimiter  RisingSlewLimit=1/(gb_shift_delay+eps)  FallingSlewLimit=-1/(gb_shift_delay+eps)
  Saturation : Saturate  UpperLimit=1  LowerLimit=0.2
  Saturation1 : Saturate  UpperLimit=gb_gears_num  LowerLimit=1
  Switch : Switch  Threshold=eps  SaturateOnIntegerOverflow=on  InputSameDT=on
  allow downshift? : Subsystem
  current gear number : Sum  SaturateOnIntegerOverflow=on
  delta gear number : Switch  Threshold=eps  SaturateOnIntegerOverflow=on  InputSameDT=on
  downshift  command : Subsystem
  engine torque capability : Lookup  InputValues=fc_map_spd*fc_spd_scale  Table=fc_max_trq*fc_trq_scale+eps  SaturateOnIntegerOverflow=on
  est eng trq : Sum  SaturateOnIntegerOverflow=on
  gb_spd_in_r : Product  SaturateOnIntegerOverflow=on
  gear ratio : Lookup  InputValues=[1:length(gb_ratio)]  Table=gb_ratio  SaturateOnIntegerOverflow=on
  gear ratio1 : Lookup  InputValues=[1:length(gb_ratio)]  Table=gb_ratio  SaturateOnIntegerOverflow=on
  gearbox speed estimator : Subsystem
  load=T/ (maxT at spd) : Saturate  UpperLimit=1  LowerLimit=0
  prev gear number : Memory  InitialCondition=gb_num_init
  prev gear ratio : Memory  InitialCondition=gb_ratio(gb_num_init)
  shifting1 : Subsystem
  upshift  command : Subsystem
  ~gb_trq_in_r : Product  Inputs=3  SaturateOnIntegerOverflow=on
  gear ratio2 : Outport  InitialOutput=0
  shifting : Outport  Port=2  InitialOutput=0
  gear number : Outport  Port=3  InitialOutput=0
  wires:
  [acc_mech_trq_est] -> est eng trq/2
  shifting1/1(out_1) -> shifting/1
  gear ratio1/1 -> gear ratio2/1
  current gear number/1 -> Saturation1/1
  Saturation/1 -> Fcn/1
  prev. Pout/Pin/1 -> Saturation/1
  gb_trq_out_r/1 -> ~gb_trq_in_r/1
  upshift  command/1(command) -> delta gear number/1, delta gear number/2
  downshift  command/1(command) -> Gain1/1
  Fcn1/1 -> ~gb_trq_in_r/3
  engine torque capability/1 -> Product2/2
  Fcn/1 -> ~gb_trq_in_r/2
  Saturation1/1 -> prev gear number/1, gear ratio1/1, gear number/1, Rate Limiter/1, shifting1/1(gear number)
  prev gear number/1 -> allow downshift?/1(prev gearnum), upshift  command/1(prev gear number), downshift  command/1(prev gear number), current gear number/1
  Product2/1 -> load=T/ (maxT at spd)/1
  Constant/1 -> Switch/1
  tires are at traction limit/1 -> Switch/2
  Rate Limiter/1 -> gear ratio/1
  gb_spd_out_r/1 -> gb_spd_in_r/1
  gb_spd_in_r/1 -> gearbox speed estimator/1(gb_spd_in_r if no gear change)
  gear ratio/1 -> prev gear ratio/1
  prev gear ratio/1 -> gb_spd_in_r/2, Fcn1/1
  Gain1/1 -> Product3/2
  Product3/1 -> delta gear number/3
  allow downshift?/1(allow shift) -> Product3/1
  gearbox speed estimator/1(Out1) -> engine torque capability/1, downshift  command/3(engine speed), upshift  command/3(engine speed)
  ~gb_trq_in_r/1 -> est eng trq/1
  est eng trq/1 -> Product2/1
  load=T/ (maxT at spd)/1 -> Switch/3
  Switch/1 -> upshift  command/2(engine load), downshift  command/2(engine load)
  delta gear number/1 -> current gear number/2

== system lib_transmission2/Gearbox Control/automatic transmission gearbox and htc advanced lock-up logic for htc shift logic for gearbox/gearbox control for use w/ AT/Block NOTES ==
  note: Lock-up of the HTC occurs when it is supposed to for the current gear, AND
      | the transmission isn't shifting, AND
      | the lockup wouldn't precipitate an immediate downshift.
  note: This gearbox control block computes the current gear number given the gearbox's
      | req'd output torque and speed and an estimate its efficiency.  Upshifts occur, given a
      | certain engine speed,  when the estimated engine load falls below the upshift curve
      | in engine speed/load space, and downshifts likewise occur when estimated engine
      | load rises above the downshift curve.  Separate upshift and downshift curves are
      | defined for each gear.  An upshift may not be immediately followed by a downshift.
      | If the tires are about to slip, don't upshift unless the engine would be at max. speed.
      | Enforce this rule by setting the load to 1 when the tires are about to slip.
